simulink model "Model2"  (R2022b)
settings: Solver=VariableStepAuto  StartTime=0.0  StopTime=10  RelTol=1e-3
undefined symbols (not defined in the file or in its folder): QAM
libraries: commrandsrc3 x1, commdigbbndam3 x1
settings Model: Creator=Ceribro  LastModifiedBy=Ceribro

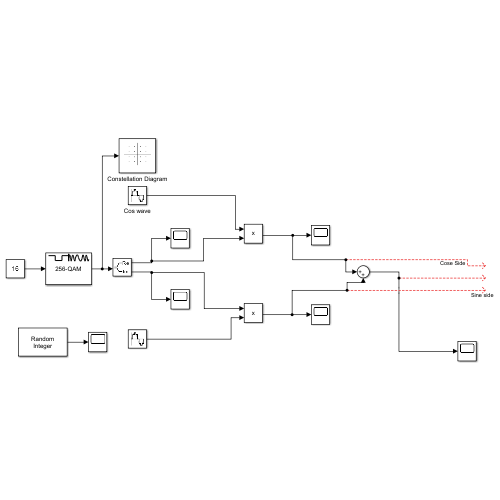
[thumbnail: Simulink's stored preview of the top-level diagram]
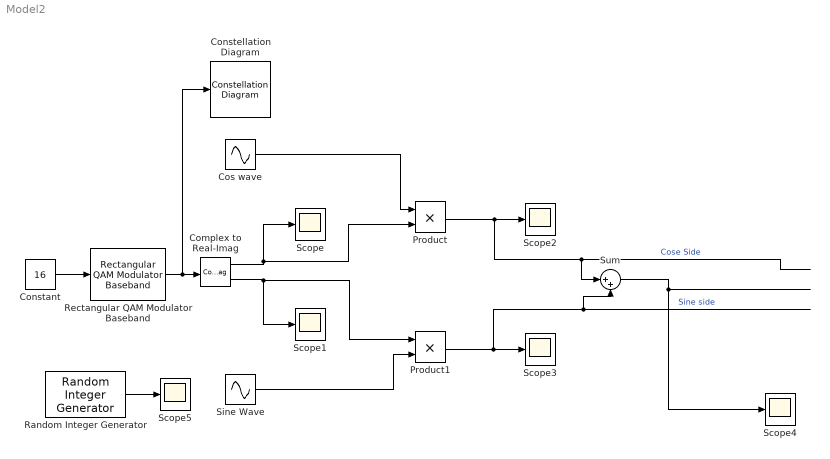
== system Model2 ==
  Complex to Real-Imag : ComplexToRealImag
  Constant : Constant  Value=16  SampleTime=0.001
  Constellation Diagram : ConstellationDiagram  WindowPosition=[382.000000,84.000000,600.000000,600.000000,]  Visible=on  ScopeFrameLocation=window  ReferenceConstellation=256-QAM  XLimits=[-15.5,15.5]  YLimits=[-15.5,15.5]  ShowLegend=on
  Cos wave : Sin  Frequency=1.257e9  Phase=pi/2  SampleTime=5e-9
  Product : Product
  Product1 : Product
  Random Integer Generator : commrandsrc3/Random Integer Generator  SetSize=256  SeedSource=Auto  Seed=0  SampleTime=0.001  SamplesPerFrame=1  OutputDataType=double  SimulateUsing=Interpreted execution
  Rectangular QAM Modulator Baseband : commdigbbndam3/Rectangular QAM Modulator Baseband  M=256  InType=Integer  Enc=Binary  Mapping=[0:15]  PowType=Min. distance between symbols  MinDist=2  AvgPow=1  PeakPow=1  Ph=0  outDtype=Fixed-point  outWordLen=16  outUDDataType=sfix(16)  outFracLenMode=User-defined  outFracLen=0  outDataTypeStr=fixdt(1,16,0)  outLastDataTypeStr=fixdt(1,16,0)
      settings: LibrarySourceBlock=|
      | commhdldigbbndam/Rectangular QAM
      | Modulator
      | Baseband
  Scope{,1..5} (6 alike) : Scope
  Sine Wave : Sin  Frequency=1.2567e9  SampleTime=5e-9
  Sum : Sum  Inputs=|++
  wires:
  Rectangular QAM Modulator Baseband/1 -> Constellation Diagram/1, Complex to Real-Imag/1
  Complex to Real-Imag/1 -> Scope/1, Product/2
  Complex to Real-Imag/2 -> Product1/1, Scope1/1
  Sine Wave/1 -> Product1/2
  Cos wave/1 -> Product/1
  Product/1 -> Sum/1, Scope2/1  "Cose Side"
  Product1/1 -> Scope3/1, Sum/2  "Sine side"
  Sum/1 -> Scope4/1
  Constant/1 -> Rectangular QAM Modulator Baseband/1
  Random Integer Generator/1 -> Scope5/1
